simulink model "lab3"  (R2015a)
settings: Solver=ode45  StartTime=0.0  StopTime=1000.0  RelTol=1e-3
values from neighbouring files (symbols this model uses):
  K = 0.08    [lab3.m]
  Ti = 200    [lab3.m]
  Toc = 3    [lab3.m]
  Tr = 1    [lab3.m]
  Ts = 16.4    [lab3.m]
  Tv = 1    [lab3.m]
settings Model: Creator=vbox  LastModifiedBy=vbox
settings DataIOCC: InspectSignalLogs=on

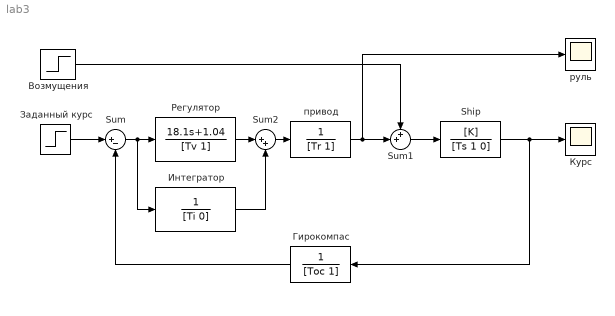
== system lab3 ==
  Ship : TransferFcn  Numerator=[K]  Denominator=[Ts 1 0]
  Sum : Sum  Inputs=|+-
  Sum1 : Sum  Inputs=++|
  Sum2 : Sum  Inputs=|++
  Возмущения : Step  After=2  SampleTime=0
  Гирокомпас : TransferFcn  Denominator=[Toc 1]
  Заданный курс : Step  Time=0  After=10  SampleTime=0
  Интегратор : TransferFcn  Numerator=1  Denominator=[Ti 0]
  Курс : Scope
      settings: SaveName=phi
  Регулятор : TransferFcn  Numerator=[18.1 1.04]  Denominator=[Tv 1]
  привод : TransferFcn  Denominator=[Tr 1]
  руль : Scope
      settings: TimeRange=100  YMin=0  YMax=400  SaveName=delta
  wires:
  Заданный курс/1 -> Sum/1
  Sum/1 -> Интегратор/1, Регулятор/1
  Гирокомпас/1 -> Sum/2
  Ship/1 -> Курс/1, Гирокомпас/1
  привод/1 -> Sum1/2, руль/1
  Возмущения/1 -> Sum1/1
  Sum1/1 -> Ship/1
  Sum2/1 -> привод/1
  Регулятор/1 -> Sum2/1
  Интегратор/1 -> Sum2/2
